simulink model "suppression_filter"  (R2013a)
settings: Solver=VariableStepDiscrete  StartTime=0.0  StopTime=60  RelTol=1e-3
InitFcn:
  | WM_Sim_config
values from neighbouring files (symbols this model uses):
  WM = WM_Sim_config(Time_length,Approx_char_rate,Tx_approx_BW,Carrier_Freq,hopping_approx_frequency,                                       hopping,Frame_len,suppression_filter,supp_filt_order,Eb_N0_dB,'noise',fec,fec_ratio)    [WM_Sim_config_smlnk_standalone.m]
libraries: dspparest3 x2, dspsrcs4 x2, dsplp x1, dspvision x1
settings Model: Creator=leonardo  LastModifiedBy=leonardo

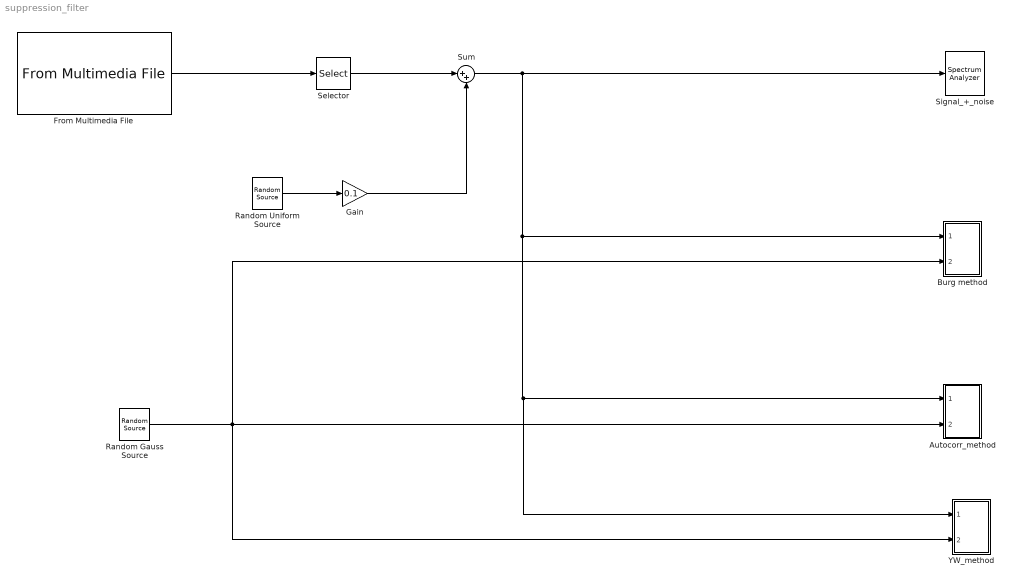
== system suppression_filter ==
  Autocorr_method : Subsystem
  Burg method : Subsystem
  From Multimedia File : dspvision/From Multimedia File  inputFilename=./audio_test/Balmorhea - Days.wav  loop=on  numPlays=1  outputStreams=Audio only  videoDataType=single  audioDataType=double  inheritSampleTime=on  userDefinedSampleTime=1/30  noAudioOutput=off  isIntensityVideo=off  fourcc=RGB  colorVideoFormat=Separate color signals  outputEOF=off  dataOrg=Column-major  audioFrameSize=WM.Sim.Frame_len  computeAudioFrameSize=off  outSamplingMode=Frame based
  Gain : Gain  Gain=0.1
  Random Gauss Source : dspsrcs4/Random Source  SrcType=Gaussian  NormMethod=Ziggurat  CltLength=12  MinVal=0  MaxVal=1  MeanVal=0  VarVal=1  RepMode=Not repeatable  rawSeed=1  IsInherit=off  SampMode=Discrete  SampTime=WM.Sim.SampleTimes.Tchannel  SampFrame=WM.Sim.Frame_len  DataType=Double  OutComplex=Real
  Random Uniform Source : dspsrcs4/Random Source  SrcType=Uniform  NormMethod=Ziggurat  CltLength=12  MinVal=-1  MaxVal=1  MeanVal=0  VarVal=1  RepMode=Not repeatable  rawSeed=1  IsInherit=off  SampMode=Discrete  SampTime=WM.Sim.SampleTimes.Tchannel  SampFrame=WM.Sim.Frame_len  DataType=Double  OutComplex=Real
  Selector : Selector  NumberOfDimensions=2  InputPortWidth=3  IndexOptions=Select all,Index vector (dialog)  Indices=[1],1  OutputSizes=1,1
  Signal_+_noise : SpectrumAnalyzer
      settings: CopyFcn=scopeextensions.ScopeBlock.callback(gcbh, 'onBlockCopy', gcbh);  DeleteFcn=scopeextensions.ScopeBlock.callback(gcbh, 'onBlockDelete');  PreSaveFcn=scopeextensions.ScopeBlock.callback(gcbh, 'onModelSave');  NameChangeFcn=scopeextensions.ScopeBlock.callback(gcbh, 'onBlockRename');  CloseFcn=scopeextensions.ScopeBlock.callback(gcbh, 'onBlockClose');  PreDeleteFcn=scopeextensions.ScopeBlock.callback(gcbh, 'onBlockPreDelete');
  Sum : Sum  Inputs=|++
  YW_method : Subsystem
  wires:
  Random Gauss Source/1 -> Burg method/2(gauss_noise_i), YW_method/2(gauss_noise_i), Autocorr_method/2(gauss_noise_i)
  Gain/1 -> Sum/2
  From Multimedia File/1 -> Selector/1
  Sum/1 -> Signal_+_noise/1, YW_method/1(signal_i), Autocorr_method/1(signal_i), Burg method/1(signal_i)
  Selector/1 -> Sum/1
  Random Uniform Source/1 -> Gain/1

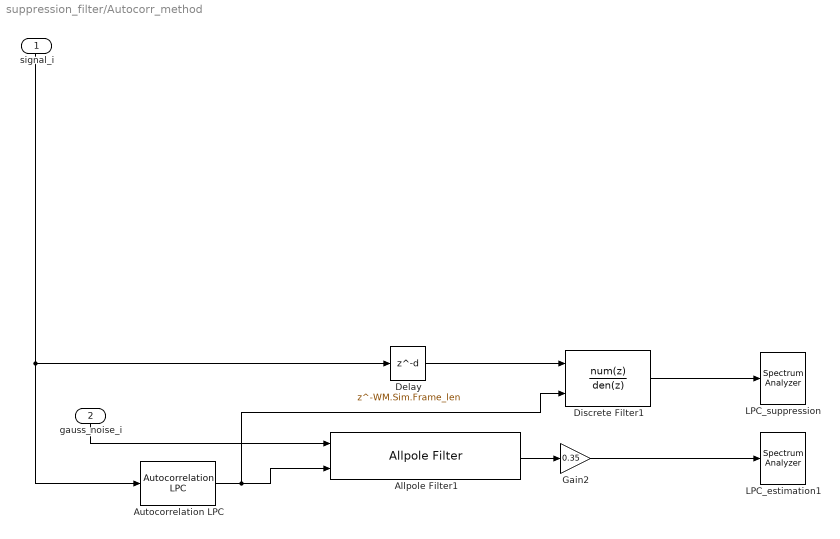
== system suppression_filter/Autocorr_method ==
  signal_i : Inport
  gauss_noise_i : Inport  Port=2
  Allpole Filter1 : AllpoleFilter  CoefSource=Input port  FilterStructure=Direct form transposed
  Autocorrelation LPC : dsplp/Autocorrelation LPC  lpcCoeffOutFcn=A  lpcOutP=off  inherit_prediction_order=off  order=WM.Sim.SuppFilt.order
  Delay : Delay  DelayLength=WM.Sim.Frame_len  InitialCondition=0  InputProcessing=Columns as channels (frame based)
  Discrete Filter1 : DiscreteFilter  NumeratorSource=Input port  Numerator=[0.5 0.5]  Denominator=[1]  InputProcessing=Columns as channels (frame based)  FilterStructure=Direct form II transposed  a0EqualsOne=on
      settings: InputPortMap=u0,p1
  Gain2 : Gain  Gain=0.35
  LPC_estimation1 : SpectrumAnalyzer
      settings: CopyFcn=scopeextensions.ScopeBlock.callback(gcbh, 'onBlockCopy', gcbh);  DeleteFcn=scopeextensions.ScopeBlock.callback(gcbh, 'onBlockDelete');  PreSaveFcn=scopeextensions.ScopeBlock.callback(gcbh, 'onModelSave');  NameChangeFcn=scopeextensions.ScopeBlock.callback(gcbh, 'onBlockRename');  CloseFcn=scopeextensions.ScopeBlock.callback(gcbh, 'onBlockClose');  PreDeleteFcn=scopeextensions.ScopeBlock.callback(gcbh, 'onBlockPreDelete');
  LPC_suppression : SpectrumAnalyzer
      settings: CopyFcn=scopeextensions.ScopeBlock.callback(gcbh, 'onBlockCopy', gcbh);  DeleteFcn=scopeextensions.ScopeBlock.callback(gcbh, 'onBlockDelete');  PreSaveFcn=scopeextensions.ScopeBlock.callback(gcbh, 'onModelSave');  NameChangeFcn=scopeextensions.ScopeBlock.callback(gcbh, 'onBlockRename');  CloseFcn=scopeextensions.ScopeBlock.callback(gcbh, 'onBlockClose');  PreDeleteFcn=scopeextensions.ScopeBlock.callback(gcbh, 'onBlockPreDelete');
  wires:
  Discrete Filter1/1 -> LPC_suppression/1
  Allpole Filter1/1 -> Gain2/1
  Autocorrelation LPC/1 -> Discrete Filter1/2, Allpole Filter1/2
  Delay/1 -> Discrete Filter1/1
  Gain2/1 -> LPC_estimation1/1
  signal_i/1 -> Autocorrelation LPC/1, Delay/1
  gauss_noise_i/1 -> Allpole Filter1/1

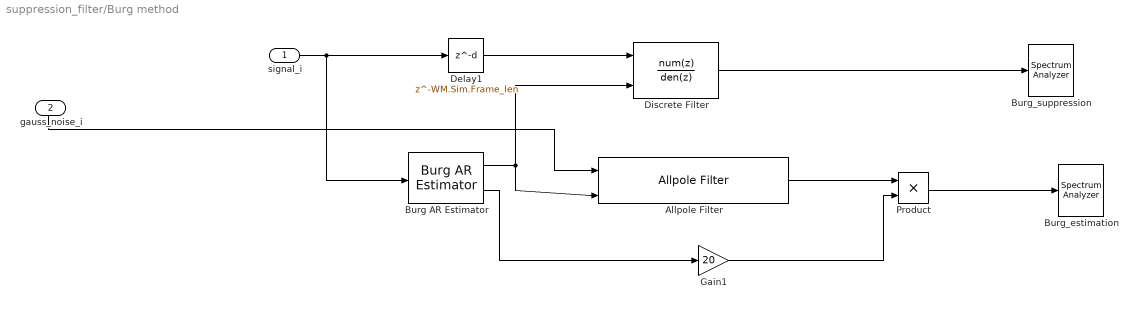
== system suppression_filter/Burg method ==
  signal_i : Inport
  gauss_noise_i : Inport  Port=2
  Allpole Filter : AllpoleFilter  CoefSource=Input port  FilterStructure=Direct form transposed
  Burg AR Estimator : dspparest3/Burg AR Estimator  fcn=A  inheritOrder=off  ord=WM.Sim.SuppFilt.order
  Burg_estimation : SpectrumAnalyzer
      settings: CopyFcn=scopeextensions.ScopeBlock.callback(gcbh, 'onBlockCopy', gcbh);  DeleteFcn=scopeextensions.ScopeBlock.callback(gcbh, 'onBlockDelete');  PreSaveFcn=scopeextensions.ScopeBlock.callback(gcbh, 'onModelSave');  NameChangeFcn=scopeextensions.ScopeBlock.callback(gcbh, 'onBlockRename');  CloseFcn=scopeextensions.ScopeBlock.callback(gcbh, 'onBlockClose');  PreDeleteFcn=scopeextensions.ScopeBlock.callback(gcbh, 'onBlockPreDelete');
  Burg_suppression : SpectrumAnalyzer
      settings: CopyFcn=scopeextensions.ScopeBlock.callback(gcbh, 'onBlockCopy', gcbh);  DeleteFcn=scopeextensions.ScopeBlock.callback(gcbh, 'onBlockDelete');  PreSaveFcn=scopeextensions.ScopeBlock.callback(gcbh, 'onModelSave');  NameChangeFcn=scopeextensions.ScopeBlock.callback(gcbh, 'onBlockRename');  CloseFcn=scopeextensions.ScopeBlock.callback(gcbh, 'onBlockClose');  PreDeleteFcn=scopeextensions.ScopeBlock.callback(gcbh, 'onBlockPreDelete');
  Delay1 : Delay  DelayLength=WM.Sim.Frame_len  InitialCondition=0  InputProcessing=Columns as channels (frame based)
  Discrete Filter : DiscreteFilter  NumeratorSource=Input port  Numerator=[0.5 0.5]  Denominator=[1]  InputProcessing=Columns as channels (frame based)  FilterStructure=Direct form II transposed  a0EqualsOne=on
      settings: InputPortMap=u0,p1
  Gain1 : Gain  Gain=20
  Product : Product
  wires:
  Allpole Filter/1 -> Product/1
  signal_i/1 -> Burg AR Estimator/1, Delay1/1
  Gain1/1 -> Product/2
  Discrete Filter/1 -> Burg_suppression/1
  Burg AR Estimator/1 -> Allpole Filter/2, Discrete Filter/2
  gauss_noise_i/1 -> Allpole Filter/1
  Delay1/1 -> Discrete Filter/1
  Burg AR Estimator/2 -> Gain1/1
  Product/1 -> Burg_estimation/1

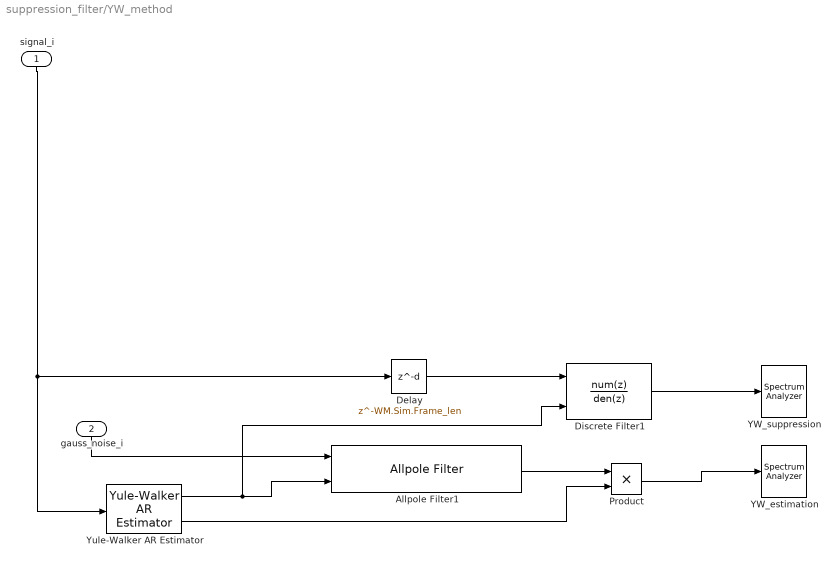
== system suppression_filter/YW_method ==
  signal_i : Inport
  gauss_noise_i : Inport  Port=2
  Allpole Filter1 : AllpoleFilter  CoefSource=Input port  FilterStructure=Direct form transposed
  Delay : Delay  DelayLength=WM.Sim.Frame_len  InitialCondition=0  InputProcessing=Columns as channels (frame based)
  Discrete Filter1 : DiscreteFilter  NumeratorSource=Input port  Numerator=[0.5 0.5]  Denominator=[1]  InputProcessing=Columns as channels (frame based)  FilterStructure=Direct form II transposed  a0EqualsOne=on
      settings: InputPortMap=u0,p1
  Product : Product
  YW_estimation : SpectrumAnalyzer
      settings: CopyFcn=scopeextensions.ScopeBlock.callback(gcbh, 'onBlockCopy', gcbh);  DeleteFcn=scopeextensions.ScopeBlock.callback(gcbh, 'onBlockDelete');  PreSaveFcn=scopeextensions.ScopeBlock.callback(gcbh, 'onModelSave');  NameChangeFcn=scopeextensions.ScopeBlock.callback(gcbh, 'onBlockRename');  CloseFcn=scopeextensions.ScopeBlock.callback(gcbh, 'onBlockClose');  PreDeleteFcn=scopeextensions.ScopeBlock.callback(gcbh, 'onBlockPreDelete');
  YW_suppression : SpectrumAnalyzer
      settings: CopyFcn=scopeextensions.ScopeBlock.callback(gcbh, 'onBlockCopy', gcbh);  DeleteFcn=scopeextensions.ScopeBlock.callback(gcbh, 'onBlockDelete');  PreSaveFcn=scopeextensions.ScopeBlock.callback(gcbh, 'onModelSave');  NameChangeFcn=scopeextensions.ScopeBlock.callback(gcbh, 'onBlockRename');  CloseFcn=scopeextensions.ScopeBlock.callback(gcbh, 'onBlockClose');  PreDeleteFcn=scopeextensions.ScopeBlock.callback(gcbh, 'onBlockPreDelete');
  Yule-Walker AR Estimator : dspparest3/Yule-Walker AR Estimator  ywArOutType=A  inheritOrder=off  ord=WM.Sim.SuppFilt.order
  wires:
  gauss_noise_i/1 -> Allpole Filter1/1
  signal_i/1 -> Yule-Walker AR Estimator/1, Delay/1
  Delay/1 -> Discrete Filter1/1
  Yule-Walker AR Estimator/1 -> Allpole Filter1/2, Discrete Filter1/2
  Discrete Filter1/1 -> YW_suppression/1
  Allpole Filter1/1 -> Product/1
  Yule-Walker AR Estimator/2 -> Product/2
  Product/1 -> YW_estimation/1
